simulink model "event_downsampler"  (R2021b)
settings: Solver=FixedStepDiscrete  StartTime=0.0  StopTime=4  FixedStep=Ts  RelTol=1e-3
model workspace (MAT data in the model file):
  Ts = Simulink.Parameter
  Ts.Value = 0.001
  Ts.Description = 'Sample time'
  Ts.DataType = 'auto'
  Ts.DocUnits = 's'
  Ts.Complexity = 'real'
  Ts.Dimensions = [1 1]
libraries: simulink x1
settings Model: Creator=upattacini  LastModifiedBy=upattacini
settings DataIOCC: SaveOutput=off  DSMLogging=off  SaveTime=off  ReturnWorkspaceOutputs=off
settings OptimizationCC: DefaultParameterBehavior=Inlined  EnhancedBackFolding=on  PassReuseOutputArgsAs=Individual arguments  ZeroExternalMemoryAtStartup=off  ZeroInternalMemoryAtStartup=off  OptimizeBlockOrder=speed  DifferentSizesBufferReuse=on  OptimizationCustomize=off  EfficientTunableParamExpr=on
settings DebuggingCC: ParameterTunabilityLossMsg=error
settings HardwareCC: ProdBitPerPointer=32  ProdBitPerSizeT=32  ProdBitPerPtrDiffT=32  ProdLargestAtomicInteger=Long  ProdLargestAtomicFloat=Double  ProdWordSize=32  ProdHWDeviceType=ARM Compatible->ARM Cortex-M
settings SFSimCC: MATLABDynamicMemAlloc=off
settings RTWCC: Description=Embedded Coder  SystemTargetFile=ert.tlc  GenCodeOnly=on  PackageGeneratedCodeAndArtifacts=on  PackageName=error_downsampler  TemplateMakefile=ert_default_tmf  TargetLang=C++
settings CodeAppCC: ForceParamTrailComments=on  IgnoreCustomStorageClasses=off  OperatorAnnotations=on  SimulinkDataObjDesc=on  SFDataObjDesc=on  InsertBlockDesc=on
settings ERTTargetCC: TargetLangStandard=C++11 (ISO)  CodeReplacementLibrary=ARM Cortex-M  GenerateSampleERTMain=on  CodeInterfacePackaging=C++ class  InlinedParameterPlacement=NonHierarchical  RootIOFormat=Structure reference  ERTCustomFileTemplate=example_file_process.tlc

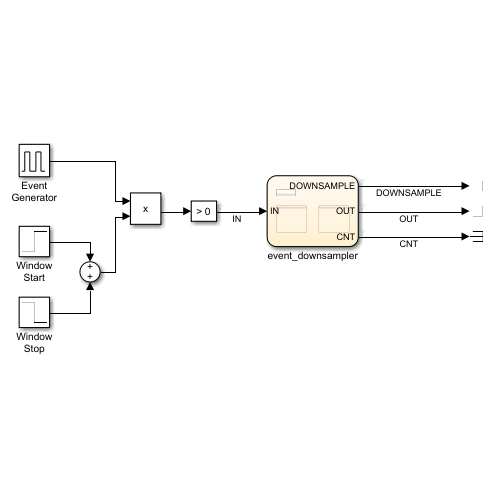
[thumbnail: Simulink's stored preview of the top-level diagram]
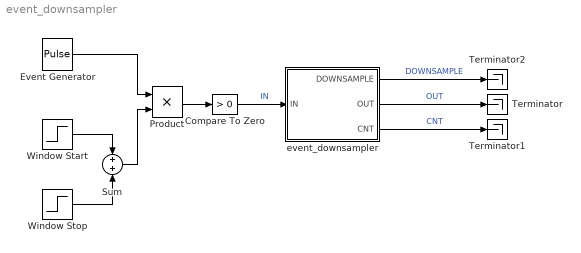
== system event_downsampler ==
  Compare To Zero : simulink/Logic and Bit Operations/Compare To Zero  relop=>  OutDataTypeStr=boolean
  Event Generator : DiscretePulseGenerator  PulseType=Time based  Period=10*Ts  PulseWidth=10
  Product : Product
  Sum : Sum
  Terminator : Terminator
  Terminator1 : Terminator
  Terminator2 : Terminator
  Window Start : Step  Time=0.1  SampleTime=0
  Window Stop : Step  Time=2.5  After=-1  SampleTime=0
  event_downsampler : Stateflow chart  TreatAsAtomicUnit=on
  wires:
  Compare To Zero/1 -> event_downsampler/1(IN)  "IN"
  event_downsampler/2(OUT) -> Terminator/1  "OUT"
  event_downsampler/3(CNT) -> Terminator1/1  "CNT"
  Window Start/1 -> Sum/1
  Window Stop/1 -> Sum/2
  Sum/1 -> Product/2
  Event Generator/1 -> Product/1
  Product/1 -> Compare To Zero/1
  event_downsampler/1(DOWNSAMPLE) -> Terminator2/1  "DOWNSAMPLE"

== stateflow chart event_downsampler/event_downsampler ==
  state EvalOccurence [parallel]
    settings: executionOrder=1
    state Run
      entry:
      acc = uint32(0);
      during, exit:
      acc = INC(IN, acc);
    (default) -> Run
    (junction 13) -> Run [order 1] : [acc < THRES_CNT]
        | /send(ev_passthrough, EventHandler)
    (junction 13) -> Run [order 2] : /send(ev_downsample, EventHandler)
    Run -> (junction 13) : after(CHECK_PER, sec)
  state EventHandler [parallel]
    settings: executionOrder=2
    state Downsample_Wait
      entry:
      DOWNSAMPLE = true;
      OUT = false;
      CNT = uint32(0);
      CNT = INC(IN, CNT);
      during, exit:
      CNT = INC(IN, CNT);
    state PassThrough
      entry, during, exit:
      DOWNSAMPLE = false;
      OUT = IN;
      CNT = INC(IN, CNT);
    state Downsample_Trigger
      entry:
      OUT = true;
      exit:
      CNT = INC(IN, CNT);
    (default) -> PassThrough
    PassThrough -> Downsample_Wait : ev_downsample
    Downsample_Trigger -> Downsample_Wait : after(1, tick)
    Downsample_Wait -> PassThrough [order 1] : ev_passthrough
    Downsample_Wait -> Downsample_Trigger [order 2] : after(CHECK_PER, sec)
  data: cond function_input boolean; in function_input uint32; out function_output uint32; acc local uint32; DOWNSAMPLE output boolean =false; OUT output boolean =false; IN input boolean; CNT output uint32 =uint32(0); THRES_CNT constant uint32 =uint32(5); CHECK_PER constant uint8 =uint8(1)
  events: ev_downsample local FUNCTION_CALL_EVENT; ev_passthrough local FUNCTION_CALL_EVENT
  function out = INC(cond, in):
    | function out = INC(cond, in)
    |  
    | if cond
    |     out = in + 1;
    | else
    |     out = in;
    | end
